simulink model "Feedback_Diversity"  (R2021a)
settings: Solver=VariableStepAuto  StartTime=0.0  StopTime=10.0  RelTol=1e-3
undefined symbols (not defined in the file or in its folder): DiscIntNeverNeededParam, doppler
libraries: commchan3 x2, commdigbbndpm3 x2
settings Model: Creator=acer  LastModifiedBy=acer

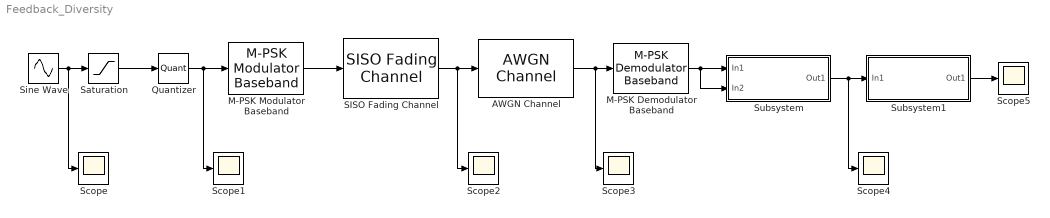
== system Feedback_Diversity ==
  AWGN Channel : commchan3/AWGN Channel  InputProcessing=Columns as channels (frame based)  seed=67  noiseMode="Signal to noise ratio  (Eb/No)"  EbNodB=10  EsNodB=10  SNRdB=10  bitsPerSym=3  Ps=1  Tsym=1  variance=1
  M-PSK Demodulator Baseband : commdigbbndpm3/M-PSK Demodulator Baseband  M=8  OutType=Integer  DecType=Hard decision  VarSource=Dialog  Variance=1  Dec=Gray  Mapping=[0:7]  Ph=pi/8  outDtype1=Inherit via internal rule  outDtype2=Inherit via internal rule  derotateFactorWordLen=16  derotateFactorDataTypeStr=Inherit: Same word length as input  derotateFactorLastDataTypeStr=Inherit: Same word length as input
  M-PSK Modulator Baseband : commdigbbndpm3/M-PSK Modulator Baseband  M=8  InType=Integer  Enc=Gray  Mapping=[0:7]  Ph=pi/8  outDtype=double  outWordLen=16  outUDDataType=sfix(16)  outFracLenMode=Best precision  outFracLen=15  outDataTypeStr=double  outLastDataTypeStr=double
  Quantizer : Quantizer  QuantizationInterval=1
  SISO Fading Channel : commchan3/SISO Fading Channel  InheritSampleRate=on  SampleRate=1  PathDelays=[0 1.5e-5]  AveragePathGains=[0 -3]  NormalizePathGains=on  FadingDistribution=Rayleigh  KFactor=3  DirectPathDopplerShift=0  DirectPathInitialPhase=0  MaximumDopplerShift=10  DopplerSpectrum=doppler('Jakes')  RandomStream=mt19937ar with seed  Seed=73  PathGainsOutputPort=off  ChannelFilterDelayOutputPort=off  SimulateUsing=Interpreted execution  Visualization=Off  PathsForDopplerDisplay=1  SamplesToDisplay=25%
  Saturation : Saturate  UpperLimit=7  LowerLimit=0
  Scope{,1..5} (6 alike) : Scope
  Sine Wave : Sin  Amplitude=3  Frequency=1000000  SampleTime=1/10000
  Subsystem : Subsystem
  Subsystem1 : Subsystem
  wires:
  Sine Wave/1 -> Scope/1, Saturation/1
  Saturation/1 -> Quantizer/1
  Quantizer/1 -> Scope1/1, M-PSK Modulator Baseband/1
  M-PSK Modulator Baseband/1 -> SISO Fading Channel/1
  SISO Fading Channel/1 -> Scope2/1, AWGN Channel/1
  AWGN Channel/1 -> Scope3/1, M-PSK Demodulator Baseband/1
  M-PSK Demodulator Baseband/1 -> Subsystem/2(In2), Subsystem/1(In1)
  Subsystem/1(Out1) -> Scope4/1, Subsystem1/1(In1)
  Subsystem1/1(Out1) -> Scope5/1

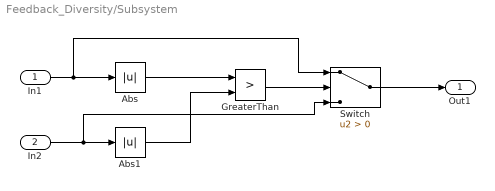
== system Feedback_Diversity/Subsystem ==
  In1 : Inport
  In2 : Inport  Port=2
  Abs : Abs
  Abs1 : Abs
  GreaterThan : RelationalOperator  Operator=>  OutDataTypeStr=boolean  RndMeth=Simplest
  Switch : Switch  Criteria=u2 > Threshold
  Out1 : Outport
  wires:
  In1/1 -> Switch/1, Abs/1
  In2/1 -> Switch/3, Abs1/1
  Abs/1 -> GreaterThan/1
  Abs1/1 -> GreaterThan/2
  GreaterThan/1 -> Switch/2
  Switch/1 -> Out1/1

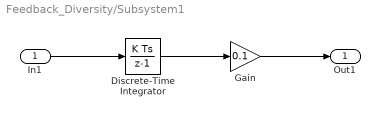
== system Feedback_Diversity/Subsystem1 ==
  In1 : Inport
  Discrete-Time Integrator : DiscreteIntegrator  SampleTime=-1  ICPrevOutput=DiscIntNeverNeededParam  ICPrevScaledInput=DiscIntNeverNeededParam
  Gain : Gain  Gain=0.1
  Out1 : Outport
  wires:
  In1/1 -> Discrete-Time Integrator/1
  Discrete-Time Integrator/1 -> Gain/1
  Gain/1 -> Out1/1
